simulink model "Figure5"  (R2021b)
settings: Solver=VariableStepAuto  StartTime=0.0  StopTime=10.0  RelTol=1e-3
undefined symbols (not defined in the file or in its folder): get, gray, res
libraries: myLib_CustomBoolean x53, dspobslib x1
settings Model: Creator=matt  LastModifiedBy=matt

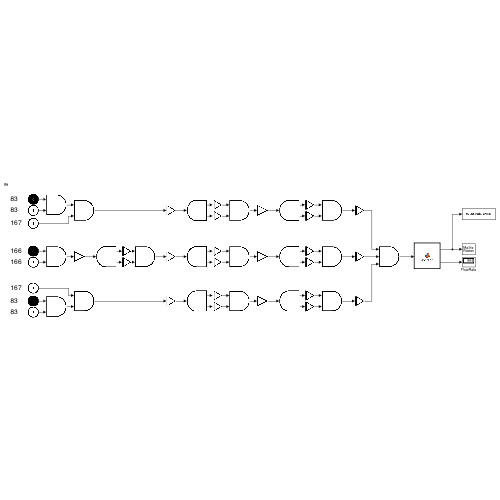
[thumbnail: Simulink's stored preview of the top-level diagram]
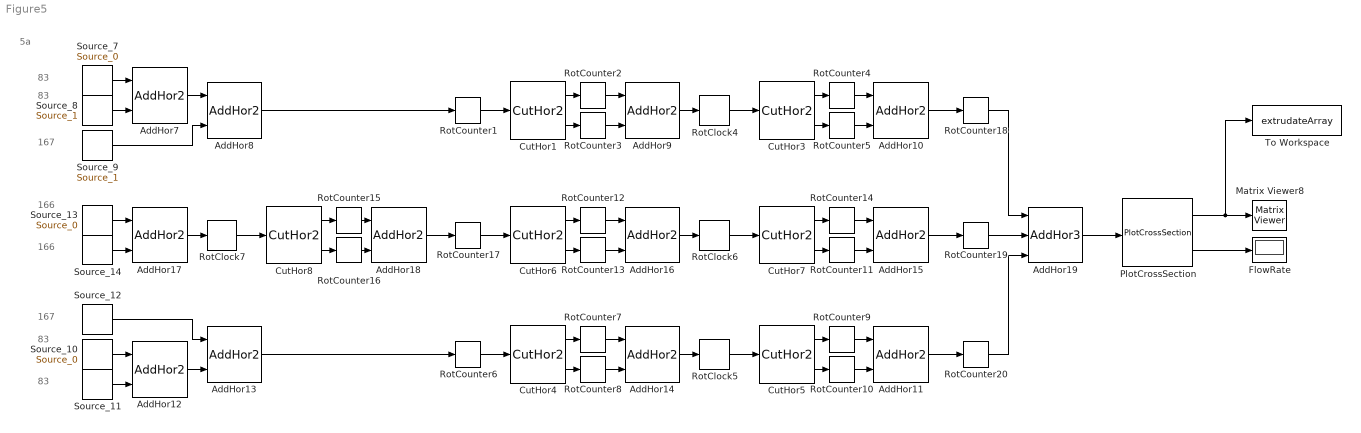
== system Figure5 ==
  note: 5a
  note: 83
  note: 166
  note: 83
  note: 167
  note: 83
  note: 166
  note: 167
  note: 83
  AddHor{7..18} (12 alike) : myLib_CustomBoolean/AddHor2  SystemSampleTime=-1  VariantActivationTime=update diagram  Latency=0  AutoFrameSizeCalculation=off
      settings: SourceProductName=Boolean_Custom_Library
  AddHor19 : myLib_CustomBoolean/AddHor3  SystemSampleTime=-1  VariantActivationTime=update diagram  Latency=0  AutoFrameSizeCalculation=off
      settings: SourceProductName=Boolean_Custom_Library
  CutHor{1,3..8} (7 alike) : myLib_CustomBoolean/CutHor2  SystemSampleTime=-1  VariantActivationTime=update diagram  Latency=0  AutoFrameSizeCalculation=off
      settings: SourceProductName=Boolean_Custom_Library
  FlowRate : Display
  Matrix Viewer8 : dspobslib/Matrix Viewer  ImageParams=off  CMapStr=gray(3)  AxisColorbar=on  AxisParams=off  AxisOrigin=Upper left corner  AxisTickMode=User-defined  XTickRange=[0 1]  YTickRange=[0 1]  XLabel=X-axis  YLabel=Y-axis  ZLabel=Z-axis  FigPos=get(0,'defaultfigureposition')  AxisZoom=off
      settings: SourceProductBaseCode=DS  YMin=0  YMax=1
  PlotCrossSection : myLib_CustomBoolean/PlotCrossSection  SystemSampleTime=-1  VariantActivationTime=update diagram  Latency=0  AutoFrameSizeCalculation=off
      settings: SourceProductName=Boolean_Custom_Library
  RotClock{4..7} (4 alike) : myLib_CustomBoolean/RotClock  SystemSampleTime=-1  VariantActivationTime=update diagram  Latency=0  AutoFrameSizeCalculation=off
      settings: SourceProductName=Boolean_Custom_Library
  RotCounter{1..20} (20 alike) : myLib_CustomBoolean/RotCounter  SystemSampleTime=-1  VariantActivationTime=update diagram  Latency=0  AutoFrameSizeCalculation=off
      settings: SourceProductName=Boolean_Custom_Library
  Source_10 : myLib_CustomBoolean/Source_0  Value=cat(3, 0.*ones(res,res), 83.*ones(res,res))  VectorParams1D=off  OutMin=[]  OutMax=[]  OutDataTypeStr=Inherit: Inherit from 'Constant value'  SampleTime=inf  FramePeriod=inf
      settings: SourceProductName=Boolean_Custom_Library
  Source_11 : myLib_CustomBoolean/Source_1  Value=cat(3, 1.*ones(res,res), 83*ones(res,res))  VectorParams1D=off  OutMin=[]  OutMax=[]  OutDataTypeStr=Inherit: Inherit from 'Constant value'  SampleTime=inf  FramePeriod=inf
      settings: SourceProductName=Boolean_Custom_Library
  Source_12 : myLib_CustomBoolean/Source_1  Value=cat(3, 1.*ones(res,res), 167*ones(res,res))  VectorParams1D=off  OutMin=[]  OutMax=[]  OutDataTypeStr=Inherit: Inherit from 'Constant value'  SampleTime=inf  FramePeriod=inf
      settings: SourceProductName=Boolean_Custom_Library
  Source_13 : myLib_CustomBoolean/Source_0  Value=cat(3, 0.*ones(res,res), 166.*ones(res,res))  VectorParams1D=off  OutMin=[]  OutMax=[]  OutDataTypeStr=Inherit: Inherit from 'Constant value'  SampleTime=inf  FramePeriod=inf
      settings: SourceProductName=Boolean_Custom_Library
  Source_14 : myLib_CustomBoolean/Source_1  Value=cat(3, 1.*ones(res,res), 166*ones(res,res))  VectorParams1D=off  OutMin=[]  OutMax=[]  OutDataTypeStr=Inherit: Inherit from 'Constant value'  SampleTime=inf  FramePeriod=inf
      settings: SourceProductName=Boolean_Custom_Library
  Source_7 : myLib_CustomBoolean/Source_0  Value=cat(3, 0.*ones(res,res), 83.*ones(res,res))  VectorParams1D=off  OutMin=[]  OutMax=[]  OutDataTypeStr=Inherit: Inherit from 'Constant value'  SampleTime=inf  FramePeriod=inf
      settings: SourceProductName=Boolean_Custom_Library
  Source_8 : myLib_CustomBoolean/Source_1  Value=cat(3, 1.*ones(res,res), 83*ones(res,res))  VectorParams1D=off  OutMin=[]  OutMax=[]  OutDataTypeStr=Inherit: Inherit from 'Constant value'  SampleTime=inf  FramePeriod=inf
      settings: SourceProductName=Boolean_Custom_Library
  Source_9 : myLib_CustomBoolean/Source_1  Value=cat(3, 1.*ones(res,res), 167*ones(res,res))  VectorParams1D=off  OutMin=[]  OutMax=[]  OutDataTypeStr=Inherit: Inherit from 'Constant value'  SampleTime=inf  FramePeriod=inf
      settings: SourceProductName=Boolean_Custom_Library
  To Workspace : ToWorkspace  VariableName=extrudateArray  SampleTime=51
  wires:
  RotCounter4/1 -> AddHor10/1
  AddHor15/1 -> RotCounter19/1
  CutHor7/2 -> RotCounter11/1
  Source_10/1 -> AddHor12/1
  RotClock6/1 -> CutHor7/1
  RotCounter13/1 -> AddHor16/2
  PlotCrossSection/2 -> FlowRate/1
  AddHor10/1 -> RotCounter18/1
  RotCounter17/1 -> CutHor6/1
  CutHor5/2 -> RotCounter10/1
  AddHor17/1 -> RotClock7/1
  RotCounter11/1 -> AddHor15/2
  Source_11/1 -> AddHor12/2
  CutHor8/1 -> RotCounter15/1
  Source_13/1 -> AddHor17/1
  RotClock7/1 -> CutHor8/1
  RotCounter3/1 -> AddHor9/2
  AddHor18/1 -> RotCounter17/1
  CutHor7/1 -> RotCounter14/1
  RotCounter16/1 -> AddHor18/2
  RotCounter15/1 -> AddHor18/1
  RotCounter9/1 -> AddHor11/1
  CutHor8/2 -> RotCounter16/1
  RotCounter18/1 -> AddHor19/1
  AddHor14/1 -> RotClock5/1
  AddHor19/1 -> PlotCrossSection/1
  CutHor6/1 -> RotCounter12/1
  RotCounter19/1 -> AddHor19/2
  AddHor12/1 -> AddHor13/2
  RotClock5/1 -> CutHor5/1
  CutHor3/2 -> RotCounter5/1
  Source_12/1 -> AddHor13/1
  CutHor3/1 -> RotCounter4/1
  CutHor6/2 -> RotCounter13/1
  CutHor4/1 -> RotCounter7/1
  RotCounter20/1 -> AddHor19/3
  AddHor9/1 -> RotClock4/1
  RotCounter6/1 -> CutHor4/1
  AddHor16/1 -> RotClock6/1
  RotCounter7/1 -> AddHor14/1
  AddHor11/1 -> RotCounter20/1
  Source_7/1 -> AddHor7/1
  RotCounter8/1 -> AddHor14/2
  Source_14/1 -> AddHor17/2
  RotCounter1/1 -> CutHor1/1
  RotCounter12/1 -> AddHor16/1
  AddHor13/1 -> RotCounter6/1
  CutHor4/2 -> RotCounter8/1
  CutHor5/1 -> RotCounter9/1
  RotClock4/1 -> CutHor3/1
  RotCounter10/1 -> AddHor11/2
  Source_9/1 -> AddHor8/2
  RotCounter5/1 -> AddHor10/2
  RotCounter2/1 -> AddHor9/1
  CutHor1/2 -> RotCounter3/1
  CutHor1/1 -> RotCounter2/1
  AddHor8/1 -> RotCounter1/1
  Source_8/1 -> AddHor7/2
  RotCounter14/1 -> AddHor15/1
  AddHor7/1 -> AddHor8/1
  PlotCrossSection/1 -> To Workspace/1, Matrix Viewer8/1
